simulink model "RLLS_Sink_Polar"  (R2013b)
settings: Solver=ode3  StartTime=0.0  StopTime=inf  FixedStep=0.025  RelTol=1e-3
InitFcn:
  | close all
  | clear all
  | clc
  | Condor_Sink_Polar_plot_2;
  | T=.025;
StopFcn:
  | Condor_Sink_Polar_plot_2_RLLS;
libraries: simulink x1, dspinverses x1
settings Model: Creator=Administrator  LastModifiedBy=vldobr
settings DebuggingCC: StateNameClashWarn=warning

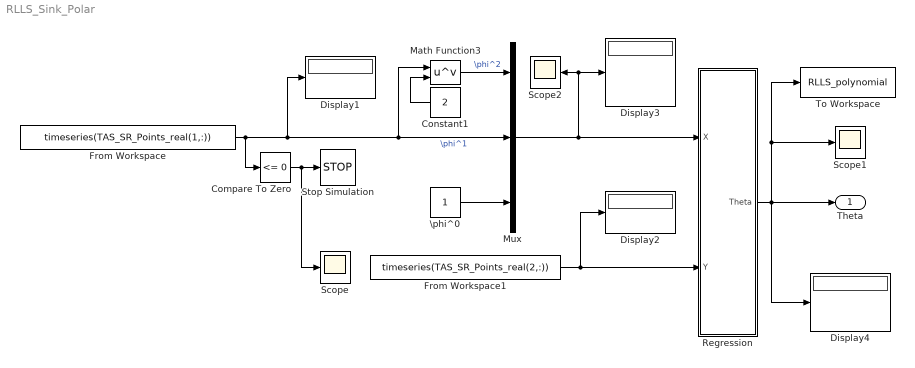
== system RLLS_Sink_Polar ==
  Compare To Zero : simulink/Logic and Bit Operations/Compare To Zero  relop=<=  OutDataTypeStr=boolean
  Constant1 : Constant  Value=2
  Display{1..4} (4 alike) : Display
  From Workspace : FromWorkspace  VariableName=timeseries(TAS_SR_Points_real(1,:))  OutputAfterFinalValue=Setting to zero
  From Workspace1 : FromWorkspace  VariableName=timeseries(TAS_SR_Points_real(2,:))  SampleTime=0
  Math Function3 : Math  Operator=pow  SaturateOnIntegerOverflow=on
  Mux : Mux  Inputs=3
  Regression : Subsystem
  Scope : Scope
  Scope1 : Scope
      settings: YMin=-0.5  YMax=5.5
  Scope2 : Scope
      settings: YMin=0  YMax=2500  SaveName=ScopeData2
  Stop Simulation : Stop
  To Workspace : ToWorkspace  VariableName=RLLS_polynomial  SampleTime=-1
  \phi^0 : Constant
  Theta : Outport
  wires:
  Regression/1(Theta) -> To Workspace/1, Scope1/1, Display4/1, Theta/1
  From Workspace1/1 -> Display2/1, Regression/2(Y)
  From Workspace/1 -> Mux/2, Math Function3/1, Display1/1, Compare To Zero/1  "\\phi^1"
  Constant1/1 -> Math Function3/2
  Compare To Zero/1 -> Scope/1, Stop Simulation/1
  Math Function3/1 -> Mux/1  "\\phi^2"
  \phi^0/1 -> Mux/3
  Mux/1 -> Scope2/1, Display3/1, Regression/1(X)

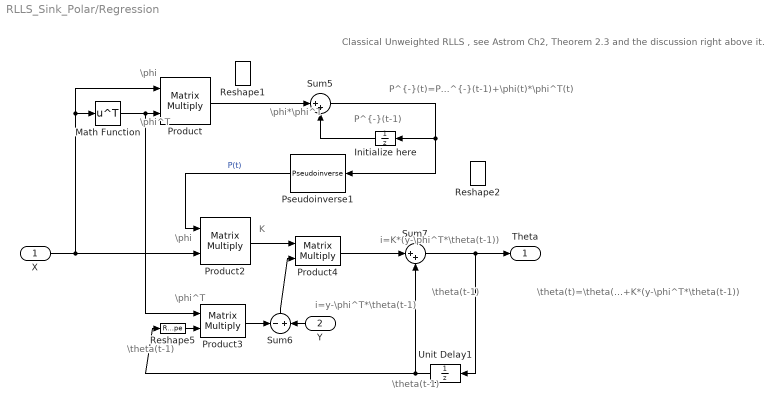
== system RLLS_Sink_Polar/Regression ==
  note: Classical Unweighted RLLS ,
      |  see Astrom Ch2, Theorem 2.3 and the discussion right above it.
  note: K
  note: P^{-}(t-1)
  note: \phi
  note: \phi*\phi^T
  note: \theta(t)=\theta(t-1)+K*(y-\phi^T*\theta(t-1))
  note: \theta(t-1)
  note: \theta(t-1)
  note: \theta(t-1)
  note: i=y-\phi^T*\theta(t-1)
  note: i=K*(y-\phi^T*\theta(t-1))
  note: P^{-}(t)=P^{-}(t-1)+\phi(t)*\phi^T(t)
  note: \phi
  note: \phi^T
  note: \phi^T
  X : Inport
  Y : Inport  Port=2
  Initialize here : UnitDelay  InitialCondition=eps*eye(3)  SampleTime=-1
  Math Function : Math  Operator=transpose  SaturateOnIntegerOverflow=on
  Product{,2..4} (4 alike) : Product  Multiplication=Matrix(*)  RndMeth=Zero
  Pseudoinverse1 : dspinverses/Pseudoinverse  wanterr=off
  Reshape1 : Reshape  OutputDimensions=[3,3]
  Reshape2 : Reshape  OutputDimensionality=Customize  OutputDimensions=[3,3]
  Reshape5 : Reshape  OutputDimensionality=Customize  OutputDimensions=[3,1]
  Sum5 : Sum  Inputs=|++  SaturateOnIntegerOverflow=on  InputSameDT=on  OutDataTypeStr=Inherit: Same as first input
  Sum6 : Sum  Inputs=-|+  SaturateOnIntegerOverflow=on  InputSameDT=on  OutDataTypeStr=Inherit: Same as first input
  Sum7 : Sum  Inputs=|++  SaturateOnIntegerOverflow=on  InputSameDT=on  OutDataTypeStr=Inherit: Same as first input
  Unit Delay1 : UnitDelay  SampleTime=T
  Theta : Outport
  wires:
  Sum5/1 -> Pseudoinverse1/1, Initialize here/1
  Product/1 -> Sum5/1
  Reshape5/1 -> Product3/2
  Initialize here/1 -> Sum5/2
  Pseudoinverse1/1 -> Product2/1  "P(t)"
  X/1 -> Product/1, Math Function/1, Product2/2
  Product2/1 -> Product4/1
  Sum6/1 -> Product4/2
  Y/1 -> Sum6/2
  Math Function/1 -> Product3/1, Product/2
  Product3/1 -> Sum6/1
  Product4/1 -> Sum7/1
  Unit Delay1/1 -> Reshape5/1, Sum7/2
  Sum7/1 -> Unit Delay1/1, Theta/1
